simulink model "EV_compensated_system_via_motor_eff_data"  (R2016a)
settings: Solver=VariableStepAuto  StartTime=0.0  StopTime=tstop  RelTol=1e-3
values from neighbouring files (symbols this model uses):
  Av = 2.16    [sim_parameters_via_motor_eff_data.m]    (also in sim_parameters_via_motor_eff_data_improved.m)
  Capacity = Capacity_cell*n_cells    (= 86939136)    [sim_parameters_via_motor_eff_data.m]    (also in sim_parameters_via_motor_eff_data_improved.m)
  Cd = 0.26    [sim_parameters_via_motor_eff_data.m]    (also in sim_parameters_via_motor_eff_data_improved.m)
  Cr = 0.01    [sim_parameters_via_motor_eff_data.m]    (also in sim_parameters_via_motor_eff_data_improved.m)
  eta_DC = .98    (= 0.98)    [sim_parameters_via_motor_eff_data.m]    (also in sim_parameters_via_motor_eff_data_improved.m)
  eta_inv = .95    (= 0.95)    [sim_parameters_via_motor_eff_data.m]    (also in sim_parameters_via_motor_eff_data_improved.m)
  Fv_max = Te_max*gratio/rw    (= 5558)    [sim_parameters_via_motor_eff_data.m]    (also in sim_parameters_via_motor_eff_data_improved.m)
  Gcm = 1000    [sim_parameters_via_motor_eff_data.m]    (also in sim_parameters_via_motor_eff_data_improved.m)
  gratio = 7.94    [sim_parameters_via_motor_eff_data.m]    (also in sim_parameters_via_motor_eff_data_improved.m)
  Ke = 0.407    [sim_parameters_via_motor_eff_data.m]    (also in sim_parameters_via_motor_eff_data_improved.m)
  motoreff_T = [0 4 8 12 16 20 24 28 32 36 40 44 ... (101 elements, 1x101)]    [MotorEff.mat]
  motoreff_w = [0 12 24 36 48 60 72 84 96 108 120 132 ... (101 elements, 1x101)]    [MotorEff.mat]
  Mv = 1250 + 55 + 15 + n_cells*weight_cell    (= 1500)    [sim_parameters_via_motor_eff_data.m]    (also in sim_parameters_via_motor_eff_data_improved.m)
  Pe_max = 80e3    (= 80000)    [sim_parameters_via_motor_eff_data.m]    (also in sim_parameters_via_motor_eff_data_improved.m)
  rho_air = 1.204    [sim_parameters_via_motor_eff_data.m]    (also in sim_parameters_via_motor_eff_data_improved.m)
  rw = 0.4    [sim_parameters_via_motor_eff_data.m]    (also in sim_parameters_via_motor_eff_data_improved.m)
  SOC_0 = 100    [sim_parameters_via_motor_eff_data.m]    (also in sim_parameters_via_motor_eff_data_improved.m)
  Te_max = 280    [sim_parameters_via_motor_eff_data.m]    (also in sim_parameters_via_motor_eff_data_improved.m)
  Vbase = Pe_max/Te_max/gratio*rw    (= 14.3936667866)    [sim_parameters_via_motor_eff_data.m]    (also in sim_parameters_via_motor_eff_data_improved.m)
  Vbat = V_cell*n_cells    (= 364.8)    [sim_parameters_via_motor_eff_data.m]    (also in sim_parameters_via_motor_eff_data_improved.m)
  Vbus_ref = 500    [sim_parameters_via_motor_eff_data.m]    (also in sim_parameters_via_motor_eff_data_improved.m)
  vref_1 = 6.7    [sim_parameters_via_motor_eff_data.m]    (also in sim_parameters_via_motor_eff_data_improved.m)
  vref_2 = 8.9    [sim_parameters_via_motor_eff_data.m]    (also in sim_parameters_via_motor_eff_data_improved.m)
  wz = 2*pi*fz    (= 1.25663706144)    [sim_parameters_via_motor_eff_data.m]    (also in sim_parameters_via_motor_eff_data_improved.m = 0.00302020992)
undefined symbols (not defined in the file or in its folder): MException, throw
libraries: simulink x4
settings Model: Creator=Gorkem  LastModifiedBy=Gorkem

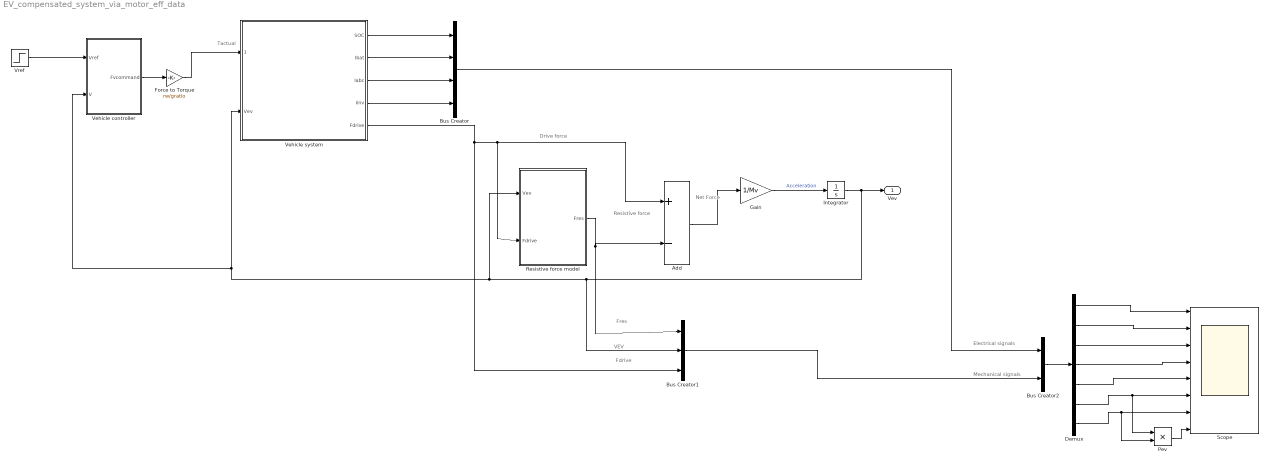
== system EV_compensated_system_via_motor_eff_data ==
  note: Fdrive
  note: VEV
  note: Fres
  note: Mechanical signals
  note: Electrical signals
  note: Resistive force
  note: Drive force
  note: Net
      | Force
  note: Tactual
  Add : Sum  Inputs=+-
  Bus Creator : BusCreator  Inputs=4
  Bus Creator1 : BusCreator  Inputs=3
  Bus Creator2 : BusCreator  Inputs=2
  Demux : Demux  Outputs=7
  Force to Torque : Gain  Gain=rw/gratio
  Gain : Gain  Gain=1/Mv
  Integrator : Integrator
  Pev : Product
  Resistive force model : Subsystem
  Scope : Scope  NumInputPorts=8
  Vehicle controller : Subsystem
  Vehicle system : Subsystem
  Vref : Step  Time=20  Before=vref_1  After=vref_2  SampleTime=0
  " Vev" : Outport
  wires:
  Add/1 -> Gain/1
  Gain/1 -> Integrator/1  "Acceleration"
  Vehicle system/5(Fdrive) -> Bus Creator1/3, Add/1, Resistive force model/2("Fdrive ")
  Resistive force model/1(Fres) -> Add/2, Bus Creator1/1
  Vehicle system/1(SOC) -> Bus Creator/1
  Vehicle system/2(Ibat) -> Bus Creator/2
  Vehicle system/3(Iabc) -> Bus Creator/3
  Vehicle system/4(Iinv) -> Bus Creator/4
  Bus Creator/1 -> Bus Creator2/1
  Bus Creator1/1 -> Bus Creator2/2
  Bus Creator2/1 -> Demux/1
  Demux/1 -> Scope/1
  Demux/2 -> Scope/2
  Demux/3 -> Scope/3
  Demux/4 -> Scope/4
  Demux/5 -> Scope/5
  Demux/6 -> Pev/1, Scope/6
  Demux/7 -> Pev/2, Scope/7
  Vref/1 -> Vehicle controller/1(Vref)
  Integrator/1 -> Bus Creator1/2, Resistive force model/1("Vev "), Vehicle system/2(Vev), Vehicle controller/2(V), " Vev"/1
  Vehicle controller/1(Fvcommand) -> Force to Torque/1
  Pev/1 -> Scope/8
  Force to Torque/1 -> Vehicle system/1(" ")

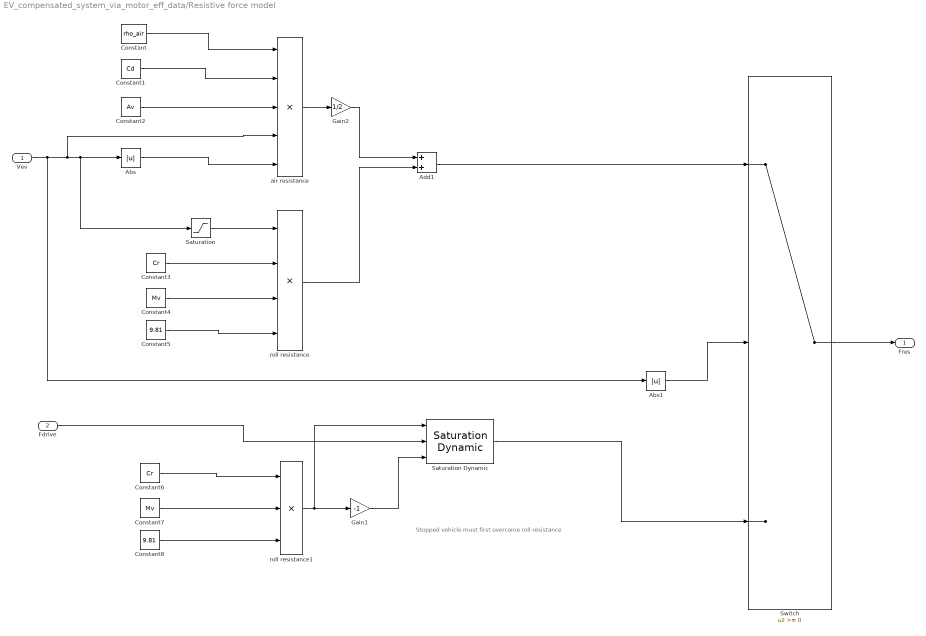
== system EV_compensated_system_via_motor_eff_data/Resistive force model ==
  note: Stopped vehicle must first overcome roll resistance
  "Vev " : Inport
  "Fdrive " : Inport  Port=2
  Abs : Abs  ZeroCross=off
  Abs1 : Abs
  Add1 : Sum
  Constant : Constant  Value=rho_air
  Constant1 : Constant  Value=Cd
  Constant2 : Constant  Value=Av
  Constant3 : Constant  Value=Cr
  Constant4 : Constant  Value=Mv
  Constant5 : Constant  Value=9.81
  Constant6 : Constant  Value=Cr
  Constant7 : Constant  Value=Mv
  Constant8 : Constant  Value=9.81
  Gain1 : Gain  Gain=-1
  Gain2 : Gain  Gain=1/2
  Saturation : Saturate  UpperLimit=1  LowerLimit=-1
  Saturation Dynamic : simulink/Discontinuities/Saturation Dynamic  OutMin=[]  OutMax=[]  OutDataTypeStr=Inherit: Same as second input  OutDataType=fixdt(1, 16)  OutScaling=2^-10  DoSatur=off
  Switch : Switch  ZeroCross=off
  "air resistance " : Product  Inputs=5
  roll resistance : Product  Inputs=4
  roll resistance1 : Product  Inputs=3
  Fres : Outport
  wires:
  Saturation Dynamic/1 -> Switch/3
  Constant2/1 -> "air resistance "/3
  Constant8/1 -> roll resistance1/3
  Gain2/1 -> Add1/1
  Constant4/1 -> roll resistance/3
  Constant1/1 -> "air resistance "/2
  Constant6/1 -> roll resistance1/1
  Constant3/1 -> roll resistance/2
  "Vev "/1 -> Abs1/1, "air resistance "/4, Saturation/1, Abs/1
  Constant/1 -> "air resistance "/1
  Constant5/1 -> roll resistance/4
  Saturation/1 -> roll resistance/1
  "air resistance "/1 -> Gain2/1
  roll resistance/1 -> Add1/2
  Constant7/1 -> roll resistance1/2
  Gain1/1 -> Saturation Dynamic/3
  Add1/1 -> Switch/1
  Abs1/1 -> Switch/2
  Switch/1 -> Fres/1
  roll resistance1/1 -> Saturation Dynamic/1, Gain1/1
  Abs/1 -> "air resistance "/5
  "Fdrive "/1 -> Saturation Dynamic/2

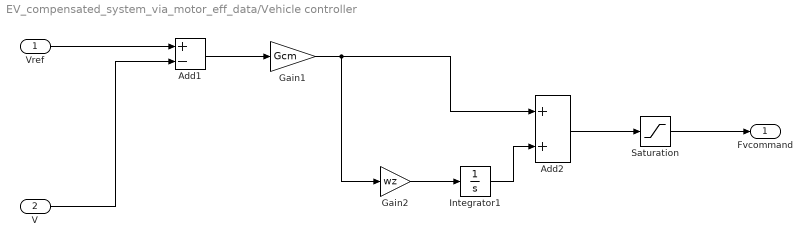
== system EV_compensated_system_via_motor_eff_data/Vehicle controller ==
  Vref : Inport
  V : Inport  Port=2
  Add1 : Sum  Inputs=+-
  Add2 : Sum
  Gain1 : Gain  Gain=Gcm
  Gain2 : Gain  Gain=wz
  Integrator1 : Integrator
  Saturation : Saturate  UpperLimit=Fv_max  LowerLimit=-Fv_max
  Fvcommand : Outport
  wires:
  Gain1/1 -> Add2/1, Gain2/1
  Gain2/1 -> Integrator1/1
  Integrator1/1 -> Add2/2
  V/1 -> Add1/2
  Add1/1 -> Gain1/1
  Add2/1 -> Saturation/1
  Vref/1 -> Add1/1
  Saturation/1 -> Fvcommand/1

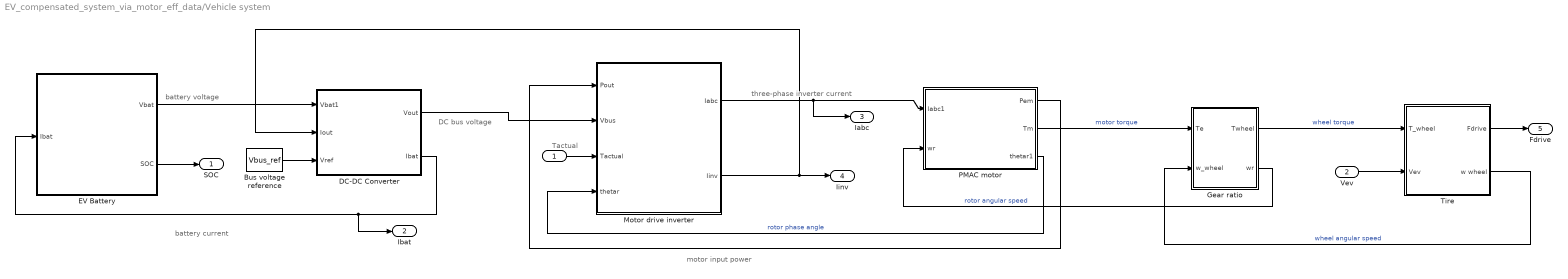
== system EV_compensated_system_via_motor_eff_data/Vehicle system ==
  note: motor input power
  note: three-phase inverter current
  note: battery current
  note: DC bus voltage
  note: Tactual
  note: battery voltage
  " " : Inport
  Vev : Inport  Port=2
  Bus voltage reference : Constant  Value=Vbus_ref
  DC-DC Converter : Subsystem
  EV Battery : Subsystem
  Gear ratio : Subsystem
  Motor drive inverter : Subsystem
  PMAC motor : Subsystem
  Tire : Subsystem
  SOC : Outport
  Ibat : Outport  Port=2
  Iabc : Outport  Port=3
  Iinv : Outport  Port=4
  Fdrive : Outport  Port=5
  wires:
  DC-DC Converter/2(Ibat) -> Ibat/1, EV Battery/1("Ibat ")
  Gear ratio/1(Twheel) -> Tire/1(T_wheel)  "wheel torque"
  " "/1 -> Motor drive inverter/3("Tactual ")
  EV Battery/1(Vbat) -> DC-DC Converter/1(Vbat1)
  PMAC motor/2(Tm) -> Gear ratio/1(Te)  "motor torque"
  DC-DC Converter/1(Vout) -> Motor drive inverter/2(Vbus)
  EV Battery/2(SOC) -> SOC/1
  Vev/1 -> Tire/2(Vev)
  Tire/2(w wheel) -> Gear ratio/2(w_wheel)  "wheel angular speed"
  Motor drive inverter/2(Iinv) -> Iinv/1, DC-DC Converter/2(Iout)
  Tire/1(Fdrive) -> Fdrive/1
  Motor drive inverter/1(Iabc) -> Iabc/1, PMAC motor/1(Iabc1)
  Bus voltage reference/1 -> DC-DC Converter/3(Vref)
  Gear ratio/2(wr) -> PMAC motor/2(wr)  "rotor angular speed"
  PMAC motor/3(thetar1) -> Motor drive inverter/4(thetar)  "rotor phase angle"
  PMAC motor/1(Pem) -> Motor drive inverter/1(Pout)

== system EV_compensated_system_via_motor_eff_data/Vehicle system/DC-DC Converter ==
  Vbat1 : Inport
  Iout : Inport  Port=2
  Vref : Inport  Port=3
  DC-DC Controller : Subsystem
  DC-DC Functional : Subsystem
  Vout : Outport
  Ibat : Outport  Port=2
  wires:
  Vbat1/1 -> DC-DC Functional/1(Vbat)
  Iout/1 -> DC-DC Functional/3(Iout)
  DC-DC Controller/1("D ") -> DC-DC Functional/2(D)
  Vref/1 -> DC-DC Controller/2(Vref)
  DC-DC Functional/1(Vout) -> Vout/1, DC-DC Controller/1(Vbus)
  DC-DC Functional/2(Ibat) -> Ibat/1

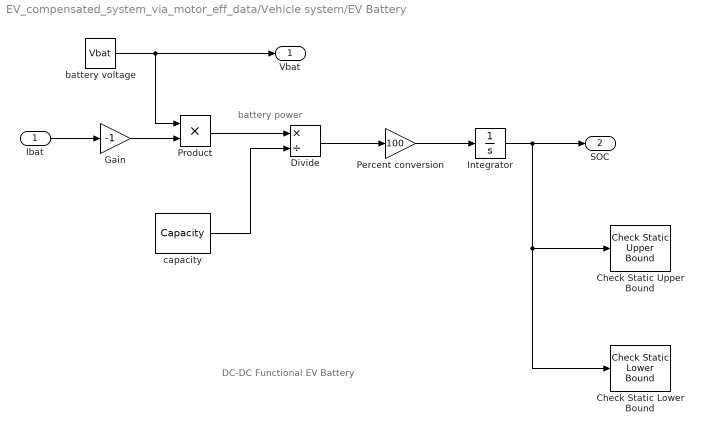
== system EV_compensated_system_via_motor_eff_data/Vehicle system/EV Battery ==
  note: DC-DC Functional EV Battery
  note: battery
      | power
  "Ibat " : Inport
  Check Static Lower Bound : simulink/Model Verification/Check Static  Lower Bound  Description=0-eps <= u  min=0-eps  min_included=on  enabled=on  callback=throw(MException('ResultChk:OutOfRange','Battery SOC has fallen below 0'))  stopWhenAssertionFail=on  export=off  icon=graphic
  Check Static Upper Bound : simulink/Model Verification/Check Static  Upper Bound  Description=u <= 100+eps  max=100+eps  max_included=on  enabled=on  callback=throw(MException('ResultChk:OutOfRange','Battery SOC has exceeded 100'))  stopWhenAssertionFail=on  export=off  icon=graphic
  Divide : Product  Inputs=*/
  Gain : Gain  Gain=-1
  Integrator : Integrator  InitialCondition=SOC_0
  Percent conversion : Gain  Gain=100
  Product : Product
  battery voltage : Constant  Value=Vbat
  capacity : Constant  Value=Capacity
  Vbat : Outport
  SOC : Outport  Port=2
  wires:
  battery voltage/1 -> Vbat/1, Product/1
  Product/1 -> Divide/1
  capacity/1 -> Divide/2
  "Ibat "/1 -> Gain/1
  Percent conversion/1 -> Integrator/1
  Divide/1 -> Percent conversion/1
  Gain/1 -> Product/2
  Integrator/1 -> SOC/1, Check Static Lower Bound/1, Check Static Upper Bound/1

== system EV_compensated_system_via_motor_eff_data/Vehicle system/Gear ratio ==
  Te : Inport
  w_wheel : Inport  Port=2
  Constant : Constant  Value=gratio
  Product : Product
  Product1 : Product
  Twheel : Outport
  wr : Outport  Port=2
  wires:
  Product/1 -> Twheel/1
  Constant/1 -> Product1/1, Product/2
  Te/1 -> Product/1
  Product1/1 -> wr/1
  w_wheel/1 -> Product1/2

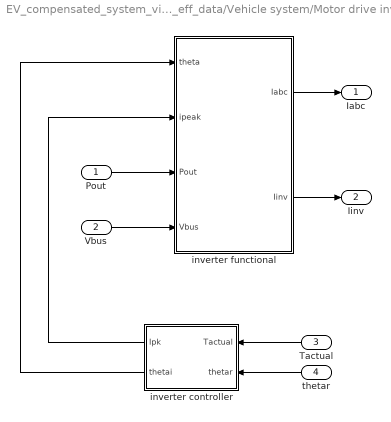
== system EV_compensated_system_via_motor_eff_data/Vehicle system/Motor drive inverter ==
  Pout : Inport
  Vbus : Inport  Port=2
  "Tactual " : Inport  Port=3
  thetar : Inport  Port=4
  inverter controller : Subsystem
  inverter functional : Subsystem
  Iabc : Outport
  Iinv : Outport  Port=2
  wires:
  inverter controller/2(thetai) -> inverter functional/1("theta ")
  inverter controller/1(Ipk) -> inverter functional/2(ipeak)
  Pout/1 -> inverter functional/3(Pout)
  inverter functional/1(Iabc) -> Iabc/1
  inverter functional/2(Iinv) -> Iinv/1
  "Tactual "/1 -> inverter controller/1("Tactual ")
  Vbus/1 -> inverter functional/4(Vbus)
  thetar/1 -> inverter controller/2(thetar)

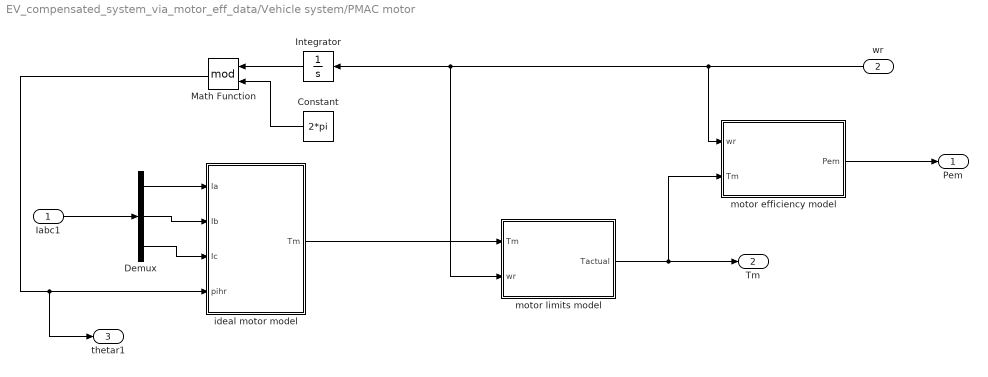
== system EV_compensated_system_via_motor_eff_data/Vehicle system/PMAC motor ==
  Iabc1 : Inport
  wr : Inport  Port=2
  Constant : Constant  Value=2*pi
  Demux : Demux  Outputs=3
  Integrator : Integrator
  Math Function : Math  Operator=mod  SaturateOnIntegerOverflow=on
  "ideal motor model " : Subsystem
  motor efficiency model : Subsystem
  motor limits model : Subsystem
  Pem : Outport
  Tm : Outport  Port=2
  thetar1 : Outport  Port=3
  wires:
  Iabc1/1 -> Demux/1
  "ideal motor model "/1(Tm) -> motor limits model/1(Tm)
  Demux/2 -> "ideal motor model "/2(Ib)
  Demux/3 -> "ideal motor model "/3(Ic)
  Integrator/1 -> Math Function/1
  motor limits model/1(Tactual) -> motor efficiency model/2(Tm), Tm/1
  motor efficiency model/1(Pem) -> Pem/1
  wr/1 -> motor efficiency model/1(wr), Integrator/1, motor limits model/2(wr)
  Constant/1 -> Math Function/2
  Demux/1 -> "ideal motor model "/1(Ia)
  Math Function/1 -> thetar1/1, "ideal motor model "/4(pihr)

== system EV_compensated_system_via_motor_eff_data/Vehicle system/Tire ==
  T_wheel : Inport
  Vev : Inport  Port=2
  Gain : Gain  Gain=1/rw
  Gain1 : Gain  Gain=1/rw
  Fdrive : Outport
  w wheel : Outport  Port=2
  wires:
  T_wheel/1 -> Gain/1
  Gain/1 -> Fdrive/1
  Vev/1 -> Gain1/1
  Gain1/1 -> w wheel/1

== system EV_compensated_system_via_motor_eff_data/Vehicle system/DC-DC Converter/DC-DC Controller ==
  Vbus : Inport
  Vref : Inport  Port=2
  Gain : Gain
  Integrator : Integrator
  Saturation : Saturate  UpperLimit=1  LowerLimit=0
  Sum : Sum  Inputs=|-+
  "D " : Outport
  wires:
  Vbus/1 -> Sum/1
  Sum/1 -> Gain/1
  Vref/1 -> Sum/2
  Gain/1 -> Integrator/1
  Integrator/1 -> Saturation/1
  Saturation/1 -> "D "/1

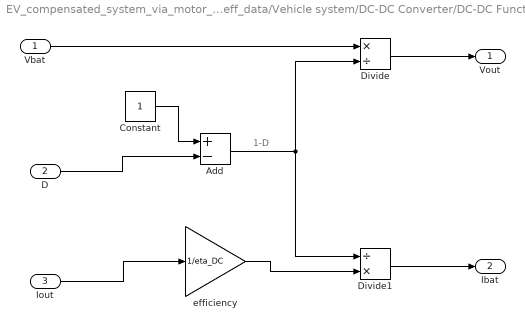
== system EV_compensated_system_via_motor_eff_data/Vehicle system/DC-DC Converter/DC-DC Functional ==
  note: 1-D
  Vbat : Inport
  D : Inport  Port=2
  Iout : Inport  Port=3
  Add : Sum  Inputs=+-
  Constant : Constant
  Divide : Product  Inputs=*/
  Divide1 : Product  Inputs=/*
  efficiency : Gain  Gain=1/eta_DC
  Vout : Outport
  Ibat : Outport  Port=2
  wires:
  Constant/1 -> Add/1
  D/1 -> Add/2
  Vbat/1 -> Divide/1
  Divide/1 -> Vout/1
  Iout/1 -> efficiency/1
  efficiency/1 -> Divide1/2
  Divide1/1 -> Ibat/1
  Add/1 -> Divide/2, Divide1/1

== system EV_compensated_system_via_motor_eff_data/Vehicle system/Motor drive inverter/inverter controller ==
  "Tactual " : Inport
  thetar : Inport  Port=2
  Torque to inverter peak current : Gain  Gain=1/Ke*2/3
  Ipk : Outport
  thetai : Outport  Port=2
  wires:
  "Tactual "/1 -> Torque to inverter peak current/1
  Torque to inverter peak current/1 -> Ipk/1
  thetar/1 -> thetai/1

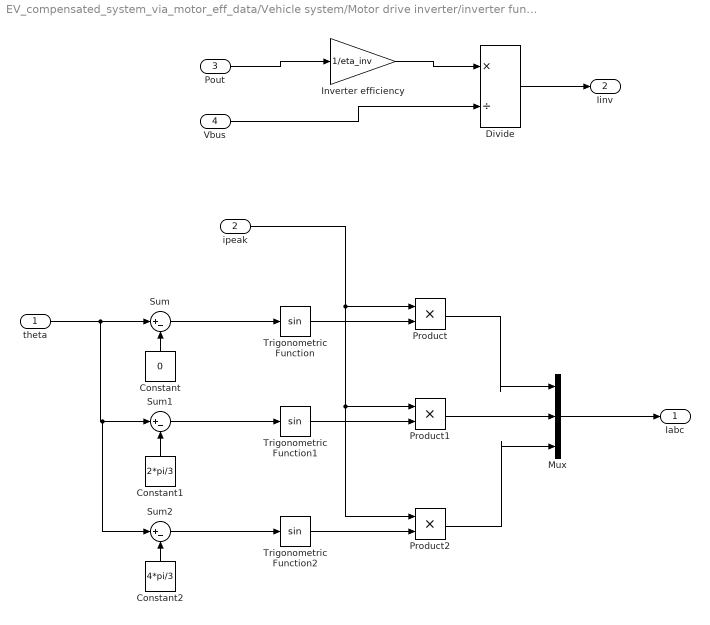
== system EV_compensated_system_via_motor_eff_data/Vehicle system/Motor drive inverter/inverter functional ==
  "theta " : Inport
  ipeak : Inport  Port=2
  Pout : Inport  Port=3
  Vbus : Inport  Port=4
  Constant : Constant  Value=0
  Constant1 : Constant  Value=2*pi/3
  Constant2 : Constant  Value=4*pi/3
  Divide : Product  Inputs=*/
  Inverter efficiency : Gain  Gain=1/eta_inv
  Mux : Mux  Inputs=3
  Product : Product
  Product1 : Product
  Product2 : Product
  Sum : Sum  Inputs=|+-
  Sum1 : Sum  Inputs=|+-
  Sum2 : Sum  Inputs=|+-
  Trigonometric Function : Trigonometry
  Trigonometric Function1 : Trigonometry
  Trigonometric Function2 : Trigonometry
  Iabc : Outport
  Iinv : Outport  Port=2
  wires:
  Constant1/1 -> Sum1/2
  Sum2/1 -> Trigonometric Function2/1
  Trigonometric Function/1 -> Product/2
  Constant2/1 -> Sum2/2
  Sum1/1 -> Trigonometric Function1/1
  Sum/1 -> Trigonometric Function/1
  "theta "/1 -> Sum2/1, Sum1/1, Sum/1
  Constant/1 -> Sum/2
  ipeak/1 -> Product2/1, Product1/1, Product/1
  Trigonometric Function2/1 -> Product2/2
  Trigonometric Function1/1 -> Product1/2
  Product1/1 -> Mux/2
  Product/1 -> Mux/1
  Product2/1 -> Mux/3
  Vbus/1 -> Divide/2
  Inverter efficiency/1 -> Divide/1
  Divide/1 -> Iinv/1
  Pout/1 -> Inverter efficiency/1
  Mux/1 -> Iabc/1

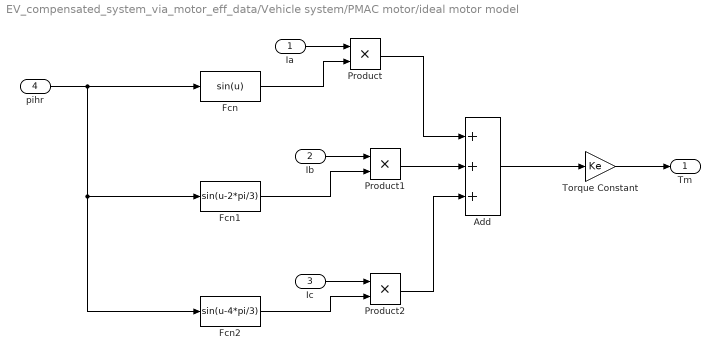
== system EV_compensated_system_via_motor_eff_data/Vehicle system/PMAC motor/ideal motor model  ==
  Ia : Inport
  Ib : Inport  Port=2
  Ic : Inport  Port=3
  pihr : Inport  Port=4
  Add : Sum  Inputs=+++
  Fcn : Fcn  Expr=sin(u)
  Fcn1 : Fcn  Expr=sin(u-2*pi/3)
  Fcn2 : Fcn  Expr=sin(u-4*pi/3)
  Product : Product
  Product1 : Product
  Product2 : Product
  Torque Constant : Gain  Gain=Ke
  Tm : Outport
  wires:
  Fcn2/1 -> Product2/2
  Ib/1 -> Product1/1
  Ia/1 -> Product/1
  Product1/1 -> Add/2
  Ic/1 -> Product2/1
  Product/1 -> Add/1
  Product2/1 -> Add/3
  Fcn/1 -> Product/2
  Add/1 -> Torque Constant/1
  Torque Constant/1 -> Tm/1
  Fcn1/1 -> Product1/2
  pihr/1 -> Fcn/1, Fcn2/1, Fcn1/1

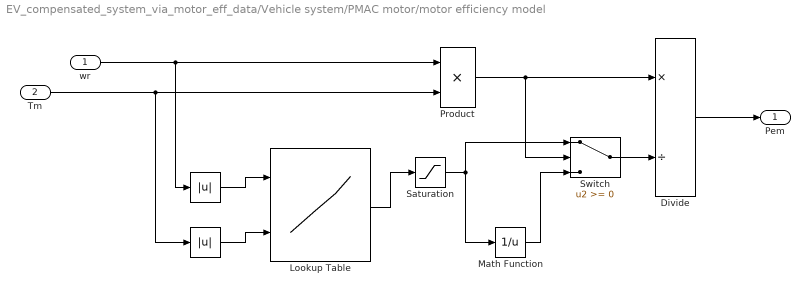
== system EV_compensated_system_via_motor_eff_data/Vehicle system/PMAC motor/motor efficiency model ==
  wr : Inport
  Tm : Inport  Port=2
  "   " : Abs
  "       " : Abs
  Divide : Product  Inputs=*/
  Lookup Table : Lookup_n-D  BreakpointsForDimension1=motoreff_w  BreakpointsForDimension2=motoreff_T  Table=motoreff'  ExtrapMethod=Clip  UseLastTableValue=on  RndMeth=Simplest  InputSameDT=on
  Math Function : Math  Operator=reciprocal  SaturateOnIntegerOverflow=on
  Product : Product  RndMeth=Zero
  Saturation : Saturate  UpperLimit=1  LowerLimit=.05
  Switch : Switch
  Pem : Outport
  wires:
  Divide/1 -> Pem/1
  "       "/1 -> Lookup Table/2
  "   "/1 -> Lookup Table/1
  Lookup Table/1 -> Saturation/1
  wr/1 -> "   "/1, Product/1
  Tm/1 -> "       "/1, Product/2
  Switch/1 -> Divide/2
  Product/1 -> Switch/2, Divide/1
  Saturation/1 -> Math Function/1, Switch/1
  Math Function/1 -> Switch/3

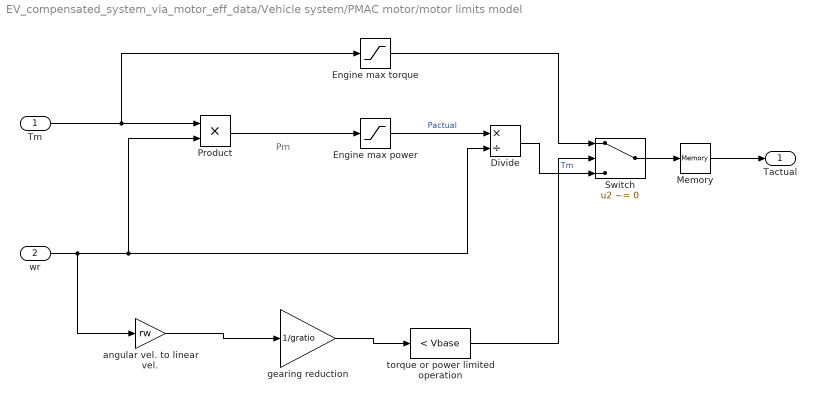
== system EV_compensated_system_via_motor_eff_data/Vehicle system/PMAC motor/motor limits model ==
  note: Pm
  Tm : Inport
  wr : Inport  Port=2
  Divide : Product  Inputs=*/
  Engine max power : Saturate  UpperLimit=Pe_max  LowerLimit=-Pe_max  ZeroCross=off
  Engine max torque : Saturate  UpperLimit=Te_max  LowerLimit=-Te_max  ZeroCross=off
  Memory : Memory
  Product : Product
  Switch : Switch  Criteria=u2 ~= 0
  angular vel. to linear vel. : Gain  Gain=rw
  gearing reduction : Gain  Gain=1/gratio
  torque or power limited operation : simulink/Logic and Bit Operations/Compare To Constant  relop=<  const=Vbase  OutDataTypeStr=boolean
  Tactual : Outport
  wires:
  Product/1 -> Engine max power/1
  Engine max torque/1 -> Switch/1
  Tm/1 -> Engine max torque/1, Product/1
  Divide/1 -> Switch/3  "Tm"
  torque or power limited operation/1 -> Switch/2
  wr/1 -> angular vel. to linear vel./1, Product/2, Divide/2
  gearing reduction/1 -> torque or power limited operation/1
  Switch/1 -> Memory/1
  Memory/1 -> Tactual/1
  Engine max power/1 -> Divide/1  "Pactual"
  angular vel. to linear vel./1 -> gearing reduction/1
